simulink model "atomnedrustning"  (R2018b)
settings: Solver=VariableStepAuto  StartTime=0.0  StopTime=100  FixedStep=0.1  RelTol=1e-3
values from neighbouring files (symbols this model uses):
  nedrustningsavtale_blanisser = 282    [parameeters.m]
  nedrustningsavtale_rodnisser = 615    [parameeters.m]
  oppdaget_atomvapen = 5    [parameeters.m]
  T1 = t    (= 1000)    [parameeters.m]
  T2 = t    (= 1000)    [parameeters.m]
  T3 = t    (= 1000)    [parameeters.m]
  T4 = t    (= 1000)    [parameeters.m]
  wish_to_be_world_police = 1    [parameeters.m]
settings Model: Creator=96andaur  LastModifiedBy=Magne Sirnes
settings DebuggingCC: LibraryContextMissingDiagnostic=none
settings SFSimCC: SimUseLocalCustomCode=off
settings RTWCC: RTWUseLocalCustomCode=off

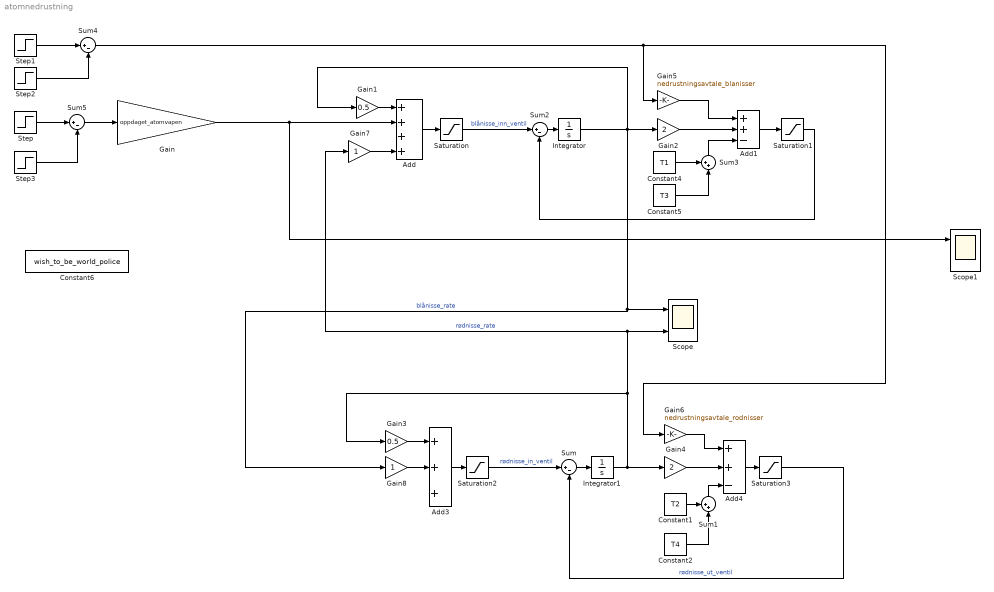
== system atomnedrustning ==
  Add : Sum  Inputs=++++
  Add1 : Sum  Inputs=++-
  Add3 : Sum  Inputs=+++
  Add4 : Sum  Inputs=++-
  Constant1 : Constant  Value=T2
  Constant2 : Constant  Value=T4
  Constant4 : Constant  Value=T1
  Constant5 : Constant  Value=T3
  Constant6 : Constant  Value=wish_to_be_world_police
  Gain : Gain  Gain=oppdaget_atomvapen
  Gain1 : Gain  Gain=0.5
  Gain2 : Gain  Gain=2
  Gain3 : Gain  Gain=0.5
  Gain4 : Gain  Gain=2
  Gain5 : Gain  Gain=nedrustningsavtale_blanisser
  Gain6 : Gain  Gain=nedrustningsavtale_rodnisser
  Gain7 : Gain
  Gain8 : Gain
  Integrator : Integrator
  Integrator1 : Integrator
  Saturation{,1..3} (4 alike) : Saturate  UpperLimit=inf  LowerLimit=0
  Scope : Scope  NumInputPorts=2
  Scope1 : Scope  NumInputPorts=2
  Step : Step  Time=38  SampleTime=0
  Step1 : Step  Time=88  SampleTime=0
  Step2 : Step  Time=91  SampleTime=0
  Step3 : Step  Time=39  SampleTime=0
  Sum{,2,4..5} (4 alike) : Sum  Inputs=|+-
  Sum1 : Sum  Inputs=++|
  Sum3 : Sum  Inputs=++|
  wires:
  Constant5/1 -> Sum3/2
  Constant4/1 -> Sum3/1
  Add/1 -> Saturation/1
  Add1/1 -> Saturation1/1
  Sum2/1 -> Integrator/1
  Saturation/1 -> Sum2/1  "blånisse_inn_ventil"
  Gain/1 -> Scope1/1, Add/2
  Sum3/1 -> Add1/3
  ? -> Add/3, Add3/3
  Integrator/1 -> Gain2/1, Gain1/1, Gain8/1, Scope/1  "blånisse_rate"
  Gain1/1 -> Add/1
  Add3/1 -> Saturation2/1
  Saturation2/1 -> Sum/1  "rødnisse_in_ventil"
  Gain4/1 -> Add4/2
  Saturation3/1 -> Sum/2  "rødnisse_ut_ventil"
  Integrator1/1 -> Gain3/1, Gain7/1, Scope/2, Gain4/1  "rødnisse_rate"
  Sum/1 -> Integrator1/1
  Add4/1 -> Saturation3/1
  Sum1/1 -> Add4/3
  Gain3/1 -> Add3/1
  Constant2/1 -> Sum1/2
  Constant1/1 -> Sum1/1
  Saturation1/1 -> Sum2/2
  Gain2/1 -> Add1/2
  Sum4/1 -> Gain6/1, Gain5/1
  Step/1 -> Sum5/1
  Sum5/1 -> Gain/1
  Step1/1 -> Sum4/1
  Step2/1 -> Sum4/2
  Gain5/1 -> Add1/1
  Gain6/1 -> Add4/1
  Step3/1 -> Sum5/2
  Gain7/1 -> Add/4
  Gain8/1 -> Add3/2
  ? -> Scope1/2
